simulink model "robot"  (R2022b)
settings: Solver=VariableStepAuto  StartTime=0.0  StopTime=10  FixedStep=0.01  RelTol=1e-3
settings Model: Creator=bassam  LastModifiedBy=bassam

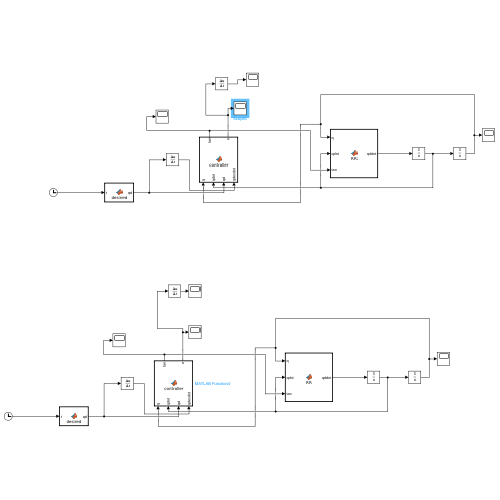
[thumbnail: Simulink's stored preview of the top-level diagram]
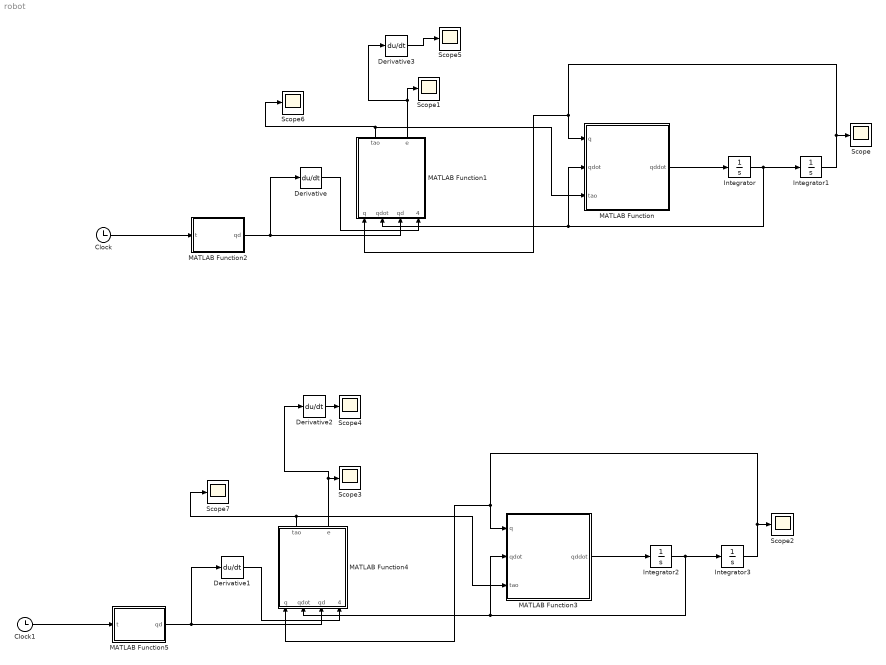
== system robot ==
  Clock : Clock
  Clock1 : Clock
  Derivative{,1..3} (4 alike) : Derivative
  Integrator{,1..3} (4 alike) : Integrator
  MATLAB Function : MATLAB Function  TreatAsAtomicUnit=on
  MATLAB Function1 : MATLAB Function  TreatAsAtomicUnit=on
  MATLAB Function2 : MATLAB Function  TreatAsAtomicUnit=on
  MATLAB Function3 : MATLAB Function  TreatAsAtomicUnit=on
  MATLAB Function4 : MATLAB Function  TreatAsAtomicUnit=on
  MATLAB Function5 : MATLAB Function  TreatAsAtomicUnit=on
  Scope{,1..7} (8 alike) : Scope
  wires:
  MATLAB Function/1(qddot) -> Integrator/1
  MATLAB Function2/1(qd) -> Derivative/1, MATLAB Function1/3(qd)
  Derivative/1 -> MATLAB Function1/4(qdesdot)
  Integrator1/1 -> Scope/1, MATLAB Function1/1(q), MATLAB Function/1(q)
  Integrator/1 -> MATLAB Function1/2(qdot), MATLAB Function/2(qdot), Integrator1/1
  Clock/1 -> MATLAB Function2/1(t)
  Integrator2/1 -> MATLAB Function4/2(qdot), MATLAB Function3/2(qdot), Integrator3/1
  MATLAB Function5/1(qd) -> Derivative1/1, MATLAB Function4/3(qd)
  Integrator3/1 -> Scope2/1, MATLAB Function4/1(q), MATLAB Function3/1(q)
  MATLAB Function3/1(qddot) -> Integrator2/1
  Derivative1/1 -> MATLAB Function4/4(qdesdot)
  Clock1/1 -> MATLAB Function5/1(t)
  MATLAB Function4/2(e) -> Derivative2/1, Scope3/1
  Derivative2/1 -> Scope4/1
  MATLAB Function1/2(e) -> Derivative3/1, Scope1/1
  Derivative3/1 -> Scope5/1
  MATLAB Function1/1(tao) -> Scope6/1, MATLAB Function/3(tao)
  MATLAB Function4/1(tao) -> Scope7/1, MATLAB Function3/3(tao)

== matlab function robot/MATLAB Function1 ==
  data: tao output; q input; qdot input; qd input; qdesdot input; e output
function [tao,e]= controller(q,qdot,qd,qdesdot)

tao = [0;0];


Kp = [25 0; 0 25];
Kd = [3 0; 0 3];


e = (qd - q);
edot = (qdesdot - qdot);



u = Kp * e + Kd*edot;





theta1 = q(1);
theta2 = q(2);
dtheta1 = qdot(1);
dtheta2 = qdot(2);

m1 = 3.473;
m2 = 0.196;
a1 = 1;
a2 = 1;
g = -9.81;
f1 = 5.3;
f2 = 1.1;
 


M = [(m1+m2)*(a1^2) + m2*(a2^2) + 2*m2*a1*a2*cos(theta1) m2*(a2^2)+m2*a1*a2*cos(theta2);
      m2*(a2)^2 + m2*a1*a2*cos(theta2) m2*a2*a2];

V = [-m2*a1*a2*(2*dtheta1*dtheta2 + dtheta2*dtheta2)*sin(theta2); m2*a1*a2*(theta1*theta1)*sin(theta2)];

F = [f1 0;0 f2];

G = [(m1+m2)*g*a1*cos(theta1)+m2*g*a2*cos(theta1+theta2); m2*g*a2*cos(theta1+theta2)];


tao = M*u + V + F *qdot + G;

== matlab function robot/MATLAB Function ==
  data: q input; qddot output; qdot input; tao input
function qddot =  RR(q,qdot,tao)

qddot = [0;0];
theta1 = q(1);
theta2 = q(2);
dtheta1 = qdot(1);
dtheta2 = qdot(2);

m1 = 3.473;
m2 = 0.196;
a1 = 1;
a2 = 1;
g = -9.81;
f1 = 5.3;
f2 = 1.1;
 


M = [(m1+m2)*(a1^2) + m2*(a2^2) + 2*m2*a1*a2*cos(theta1) m2*(a2^2)+m2*a1*a2*cos(theta2);
      m2*(a2)^2 + m2*a1*a2*cos(theta2) m2*a2*a2];

V = [-m2*a1*a2*(2*dtheta1*dtheta2 + dtheta2*dtheta2)*sin(theta2); m2*a1*a2*(theta1*theta1)*sin(theta2)];

F = [f1 0;0 f2];

G = [(m1+m2)*g*a1*cos(theta1)+m2*g*a2*cos(theta1+theta2); m2*g*a2*cos(theta1+theta2)];

m_inv = inv(M);

qddot =  m_inv*(tao - (V + F*qdot + G))

== matlab function robot/MATLAB Function2 ==
  data: t input; qd output
function qd = desired(t)

qd = [pi/3 + pi/6 *sin(t);pi/4 + pi/6 * cos(t)];

== matlab function robot/MATLAB Function3 ==
  data: q input; qddot output; qdot input; tao input
function qddot =  RR(q,qdot,tao)

qddot = [0;0];
theta1 = q(1);
theta2 = q(2);
dtheta1 = qdot(1);
dtheta2 = qdot(2);

m1 = 3.473;
m2 = 0.196;
a1 = 1;
a2 = 1;
g = -9.81;
f1 = 5.3;
f2 = 1.1;
 


M = [(m1+m2)*(a1^2) + m2*(a2^2) + 2*m2*a1*a2*cos(theta1) m2*(a2^2)+m2*a1*a2*cos(theta2);
      m2*(a2)^2 + m2*a1*a2*cos(theta2) m2*a2*a2];

V = [-m2*a1*a2*(2*dtheta1*dtheta2 + dtheta2*dtheta2)*sin(theta2); m2*a1*a2*(theta1*theta1)*sin(theta2)];

F = [f1 0;0 f2];

G = [(m1+m2)*g*a1*cos(theta1)+m2*g*a2*cos(theta1+theta2); m2*g*a2*cos(theta1+theta2)];

m_inv = inv(M);

qddot =  m_inv*(tao - (V + F*qdot + G))

== matlab function robot/MATLAB Function4 ==
  data: tao output; q input; qdot input; qd input; qdesdot input; e output
function [tao,e]= controller(q,qdot,qd,qdesdot)

tao = [0;0];


Kp = [25 0; 0 25];
Kd = [3 0; 0 3];


e = (qd - q);
edot = (qdesdot - qdot);



tao = Kp * e + Kd*edot;

== matlab function robot/MATLAB Function5 ==
  data: t input; qd output
function qd = desired(t)

qd = [pi/3 + pi/6 *sin(t);pi/4 + pi/6 * cos(t)];
